simulink model "FourWheelSim_base"  (R2021b)
settings: Solver=ode4  StartTime=0.0  StopTime=100  FixedStep=0.001  EnableMultiTasking=on
values from neighbouring files (symbols this model uses):
  a_f = [1.434106444513048,-3.490394354141787e-04,2.761516722659314,6.000050177239062e+04,2.990012596710455e+03,-1.736376596503330e-04,0.526021936511837]    [VehicleParams20_ver230707.m]
  a_r = a_f    [VehicleParams20_ver230707.m]
  afx_f = [1.736519934348130,-2.903281841026900e-04,2.651682004580759,7.000047010028531e+04,3.270011055825476e+03,-0.001252141095807,1.596836353939939]    [VehicleParams20_ver230707.m]
  afx_r = afx_f    [VehicleParams20_ver230707.m]
  agx_f = [0.230000000000000,2.936116597489246e+04,7.137436879966481e+03,0,0]    [VehicleParams20_ver230707.m]
  agx_r = agx_f    [VehicleParams20_ver230707.m]
  agy_f = [0.852564208514954,3.000069064154418e+04,2.070023877794581e+03,-5.089267464508360e-04,0.519364283925805]    [VehicleParams20_ver230707.m]
  agy_r = agy_f    [VehicleParams20_ver230707.m]
  b_f = [3.436650779629654,1.566044221042620e-05,0.028598122547093,3.408741969645286e+03,5.995144285148312e+03,-1.736376595720277e-04,0.526021936449385]    [VehicleParams20_ver230707.m]
  Brake_Factor = 0.66    [VehicleParams20_ver230707.m]
  Cd = Cd/(40/3.6)^2    (= 0.6885)    [VehicleParams20_ver230707.m]
  CLF = DFf/40/40    (= 0.06)    [VehicleParams20_ver230707.m]
  CLR = DFr/40/40    (= 0.065)    [VehicleParams20_ver230707.m]
  cPiston_Area_F = 2*pi*(0.0254/2)^2    (= 0.00101341495819)    [VehicleParams20_ver230707.m]
  cPiston_Area_R = 2*pi*(0.0254/2)^2    (= 0.00101341495819)    [VehicleParams20_ver230707.m]
  delta = 15.5    [VehicleParams20_ver230707.m]
  df = 1.225    [VehicleParams20_ver230707.m]
  dr = 1.225    [VehicleParams20_ver230707.m]
  eff_Radius_F = (180/2-13.5)/1000    (= 0.0765)    [VehicleParams20_ver230707.m]
  eff_Radius_R = (180/2-13.5)/1000    (= 0.0765)    [VehicleParams20_ver230707.m]
  Fd = 60*2    (= 120)    [VehicleParams20_ver230707.m]
  Frtoe = 0    [VehicleParams20_ver230707.m]
  gear_f = 13.75    [VehicleParams20_ver230707.m]
  gear_r = 13.75    [VehicleParams20_ver230707.m]
  hg = 0.28    [VehicleParams20_ver230707.m]
  HV_voltage = 600    [VehicleParams20_ver230707.m]
  I = 112    [VehicleParams20_ver230707.m]
  ini_v = ini_speed/3.6    (= 10.4166666667)    [VehicleParams20_ver230707.m]
  Kframe = 5.94*10^6    (= 5940000)    [VehicleParams20_ver230707.m]
  kk_f = 2800*180/pi    (= 160428.182637)    [VehicleParams20_ver230707.m]
  kk_r = 4200*180/pi    (= 240642.273955)    [VehicleParams20_ver230707.m]
  krfr = 0.5    [VehicleParams20_ver230707.m]
  l = 1.530    (= 1.53)    [VehicleParams20_ver230707.m]
  lf = l*(1-WBf)    (= 0.7956)    [VehicleParams20_ver230707.m]
  lr = l*WBf    (= 0.7344)    [VehicleParams20_ver230707.m]
  M = 200+60    (= 260)    [VehicleParams20_ver230707.m]
  mu_tire_F = 0.587-0.587+0.55    (= 0.55)    [VehicleParams20_ver230707.m]
  mu_tire_R = 0.587-0.587+0.55    (= 0.55)    [VehicleParams20_ver230707.m]
  Mwf = Iwf/Rwf/Rwf    (= 3.82716814816)    [VehicleParams20_ver230707.m]
  Mwr = Iwr/Rwr/Rwr    (= 3.82716814816)    [VehicleParams20_ver230707.m]
  rcf = 0.000    (= 0)    [VehicleParams20_ver230707.m]
  rch = rcf*WBf+rcr*(1-WBf)    (= 0)    [VehicleParams20_ver230707.m]
  rcr = 0.000    (= 0)    [VehicleParams20_ver230707.m]
  Reartoe = -2    [VehicleParams20_ver230707.m]
  Rr_toe = Reartoe*pi/180    (= -0.0349065850399)    [VehicleParams20_ver230707.m]
  Rwf = 18*(25.4/1000)/2    (= 0.2286)    [VehicleParams20_ver230707.m]
  Rwr = 18*(25.4/1000)/2    (= 0.2286)    [VehicleParams20_ver230707.m]
  T_TireF = TireL_f/V    (= 0.036760000032)    [VehicleParams20_ver230707.m]
  T_TireR = TireL_r/V    (= 0.036760000032)    [VehicleParams20_ver230707.m]
  tspeed = 37.5    [VehicleParams20_ver230707.m]
  WBf = 0.48    [VehicleParams20_ver230707.m]
  zc_f = castrail_Fr/1000    (= 0)    [VehicleParams20_ver230707.m]
  zc_r = castrail_Rr/1000    (= 0)    [VehicleParams20_ver230707.m]
libraries: simulink x25, dspstat3 x1
(part 4 of 4)

== stateflow chart FourWheelSim_base/Driver/Chart ==
  note: アンダーステアのみ考慮しているので，
      | 旋回半径が小さいときは速度を大きくし，
      | 大きいときは速度を小さくする．
      | シミュレーション時間を減らすには，
      | 旋回半径がパイロンタッチギリギリになる初速にする．
      |
      | 舵角は切り増すことのみ想定しているので，
      | 初期値はなるべく小さくする．
      | 小さすぎるとシミュレーション時間が伸びるので適度に．
  state Hold0
  state Hold
    entry:
    holdCnt = holdCnt + 0.1;
  state Divergence
    entry:
    Div = 1;
  state SteerUp
    entry:
    holdCnt = 0;
    deltapre = delta;
    Rpre = R;
    during:
    delta = delta + 0.1*0.001;
  state Accel
    entry:
    holdCnt = 0;
    deltaopt = 0;
    during:
    tspeed = tspeed + 0.1*0.001;
  state Decel
    entry:
    holdCnt = 0;
    deltaopt = 0;
    during:
    tspeed = tspeed - 0.1*0.001;
  state HoldAcc
  state HoldDec
  state HoldSteer
  state SteerDown
    entry:
    delta = deltapre;
    exit:
    deltaopt = delta;
  state DecOptimum
    entry:
    tspeedopt = tspeed;
  state AccOptimum
    entry:
    tspeedopt = tspeed;
  state Optimumized
    entry:
    Vopt = tspeedopt;
  (default) -> Hold0
  Hold0 -> (junction 42) : after(10,sec)
  Hold -> (junction 42) : after(0.1,sec)
  (junction 42) -> Hold [order 3]
  (junction 42) -> Divergence [order 1] : % シミュレーション開始から20秒経過しても
      | % 定常状態にならない場合
      | [holdCnt >= 10]
  SteerDown -> (junction 42) : after(0.1,sec)
  AccOptimum -> (junction 42) : after(0.1,sec)
  DecOptimum -> (junction 42) : after(0.1,sec)
  (junction 42) -> (junction 43) [order 2] : % 定常状態になった場合
      | [abs(Vnow - tspeed) <= eV && ...
      |  Vnow - Vpre1 <= edV && ...
      |  Vnow - Vpre05 <= edV]
  (junction 43) -> (junction 162) [order 2] : % パイロンタッチがある場合
      | [Rf <= 7.625 || Rr <= 7.625]
  (junction 43) -> (junction 164) [order 3]
  (junction 162) -> Accel
  (junction 43) -> Decel [order 1] : % 旋回半径が過大の場合
      | [Rf > 7.625 + 0.05 && Rr > 7.625 + 0.05]
  (junction 164) -> SteerUp
  (junction 112) -> SteerUp
  (junction 176) -> Decel
  (junction 138) -> Accel
  Decel -> HoldDec : after(1,sec)
  Accel -> HoldAcc : after(1,sec)
  SteerUp -> HoldSteer : after(1,sec)
  (junction 106) -> HoldSteer [order 2]
  (junction 140) -> HoldAcc [order 2]
  (junction 171) -> HoldDec [order 2]
  HoldAcc -> (junction 140) : after(0.1,sec)
  HoldDec -> (junction 171) : after(0.1,sec)
  HoldSteer -> (junction 106) : after(0.1,sec)
  (junction 171) -> (junction 180) [order 1] : % 定常状態になった場合
      | [abs(Vnow - tspeed) <= eV && ...
      |  Vnow - Vpre1 <= edV && ...
      |  Vnow - Vpre05 <= edV]
  (junction 106) -> (junction 111) [order 1] : % 定常状態になった場合
      | [abs(Vnow - tspeed) <= eV && ...
      |  Vnow - Vpre1 <= edV && ...
      |  Vnow - Vpre05 <= edV]
  (junction 140) -> (junction 134) [order 1] : % 定常状態になった場合
      | [abs(Vnow - tspeed) <= eV && ...
      |  Vnow - Vpre1 <= edV && ...
      |  Vnow - Vpre05 <= edV]
  (junction 180) -> (junction 176) [order 1] : % 旋回半径が過大の場合
      | [Rf > 7.625 + 0.05 && Rr > 7.625 + 0.05]
  (junction 111) -> (junction 156) [order 2] : % パイロンタッチなしかつ
      | % 舵角が最適値
      | [R > Rpre && ...
      |  deltapre == deltaopt]
  (junction 111) -> (junction 112) [order 1] : % 旋回半径が減少した場合
      | [R < Rpre]
  (junction 180) -> (junction 177) [order 2]
  (junction 134) -> (junction 138) [order 1] : % パイロンタッチがある場合
      | [Rf <= 7.625 || Rr <= 7.625]
  (junction 156) -> Optimumized
  (junction 111) -> (junction 152) [order 3]
  (junction 134) -> (junction 149) [order 2]
  (junction 177) -> DecOptimum
  (junction 152) -> SteerDown
  (junction 149) -> AccOptimum
  data: R input; Rf input; Rr input; Vnow input; Vpre1 input; tspeed output =tspeed; delta output =delta; Vopt output =0; holdCnt local =0; Rpre local; deltapre local; deltaopt local =0; tspeedopt local; Div output =0; eV constant double =1*10^-1; edV constant double =5*10^-3; Vpre05 input
